simulink model "clap_clap_on_off_arduino_nano_R2022a_Windows_DESKTOP-48TC27M_7-07-030036-2022_CaseConflict"  (R2022a)
settings: Solver=FixedStepAuto  StartTime=0.0  StopTime=inf  FixedStep=0.005  RelTol=1e-3  EnableMultiTasking=on
libraries: arduinolib x4, simulink_extras x1, eeGeneralControl x1
settings Model: ExtModeTrigDuration=2  Creator=byoun  LastModifiedBy=byoun
settings OptimizationCC: EnhancedBackFolding=on  PassReuseOutputArgsAs=Individual arguments  ZeroExternalMemoryAtStartup=off  ZeroInternalMemoryAtStartup=off  MaxStackSize=64  OptimizeBlockOrder=speed  DifferentSizesBufferReuse=on  OptimizationCustomize=off  EfficientTunableParamExpr=on
settings DebuggingCC: ParameterTunabilityLossMsg=error
settings HardwareCC: ProdBitPerInt=16  ProdBitPerPointer=16  ProdBitPerSizeT=16  ProdBitPerPtrDiffT=16  ProdLargestAtomicFloat=None  ProdWordSize=8  ProdHWDeviceType=Atmel->AVR
settings SFSimCC: MATLABDynamicMemAlloc=off
settings RTWCC: SystemTargetFile=ert.tlc  HardwareBoard=Arduino Nano 3.0  TemplateMakefile=ert_default_tmf  Toolchain=Arduino AVR  BuildConfiguration=Faster Runs
settings CodeAppCC: ForceParamTrailComments=on  IgnoreCustomStorageClasses=off  OperatorAnnotations=on  SimulinkDataObjDesc=on  SFDataObjDesc=on  InsertBlockDesc=on
settings ERTTargetCC: SupportContinuousTime=on  SupportVariableSizeSignals=on  ExtModeTransport=3  ExtModeStaticAlloc=on  ExtModeStaticAllocSize=250  ExtModeMexFile=ext_xcp  ExtModeIntrfLevel=Level2 - Open

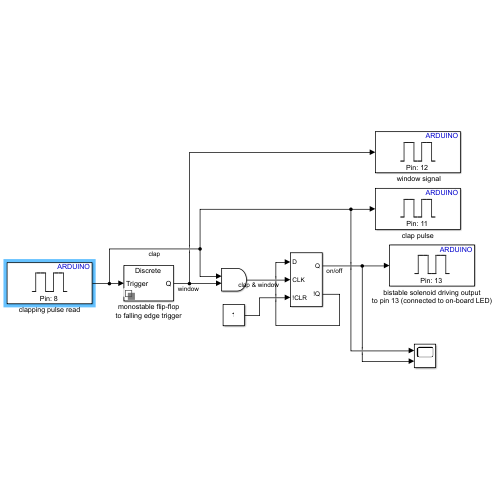
[thumbnail: Simulink's stored preview of the top-level diagram]
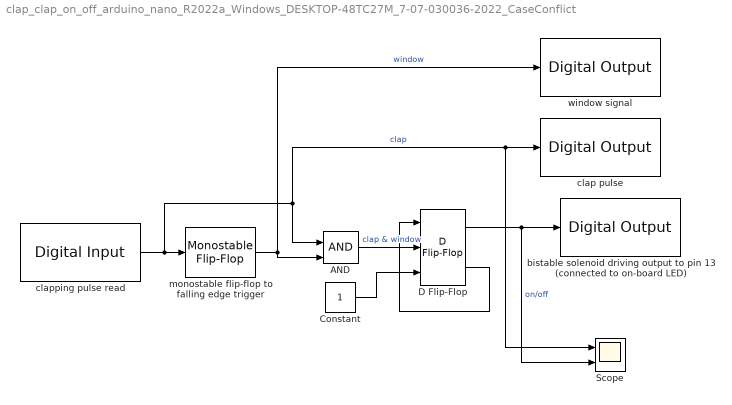
== system clap_clap_on_off_arduino_nano_R2022a_Windows_DESKTOP-48TC27M_7-07-030036-2022_CaseConflict ==
  " window signal" : arduinolib/Digital Output  pinNumber=12  Direction=output  blockPlatform=arduino
  AND : Logic  IconShape=distinctive  AllPortsSameDT=off  OutDataTypeStr=boolean
  Constant : Constant
  D Flip-Flop : simulink_extras/Flip Flops/D Flip-Flop
  Scope : Scope  NumInputPorts=2
  bistable solenoid driving output to pin 13 (connected to on-board LED) : arduinolib/Digital Output  pinNumber=13  Direction=output  blockPlatform=arduino
  clap pulse : arduinolib/Digital Output  pinNumber=11  Direction=output  blockPlatform=arduino
  clapping pulse read : arduinolib/Digital Input  pinNumber=8  mode=Default  Direction=input  SampleTime=0.01  blockPlatform=arduino
  monostable flip-flop to falling edge trigger : eeGeneralControl/Monostable Flip-Flop  VariantControl=Variant1  LabelModeActiveChoice=Discrete  ChangeType=Falling edge  x0=0  Td=0.4  Ts=0.01
      settings: SourceProductBaseCode=PS
  wires:
  clapping pulse read/1 -> AND/1, Scope/1, clap pulse/1, monostable flip-flop to falling edge trigger/1  "clap"
  monostable flip-flop to falling edge trigger/1 -> AND/2, " window signal"/1  "window"
  AND/1 -> D Flip-Flop/2  "clap & window"
  D Flip-Flop/2 -> D Flip-Flop/1
  Constant/1 -> D Flip-Flop/3
  D Flip-Flop/1 -> Scope/2, bistable solenoid driving output to pin 13 (connected to on-board LED)/1  "on/off"
